simulink model "APP_MyApplication"  (R2018b)
settings: Solver=VariableStepDiscrete  StartTime=0.0  StopTime=10  RelTol=1e-3
PreLoadFcn:
  | if(exist('MBDS_ModelCallback', 'file')), MBDS_ModelCallback('PreLoad'); end;
PostLoadFcn:
  | if(exist('MBDS_ModelCallback', 'file')), MBDS_ModelCallback('PostLoad'); end;
InitFcn:
  | if(exist('MBDS_ModelCallback', 'file')), MBDS_ModelCallback('Init'); end;
StartFcn:
  | if(exist('MBDS_ModelCallback', 'file')), MBDS_ModelCallback('Start'); end;
StopFcn:
  | if(exist('MBDS_ModelCallback', 'file')), MBDS_ModelCallback('Stop'); end;
undefined symbols (not defined in the file): sigbuilder_block, Ts
libraries: KIBES_Signal x499, simulink x8
(part 7 of 10)

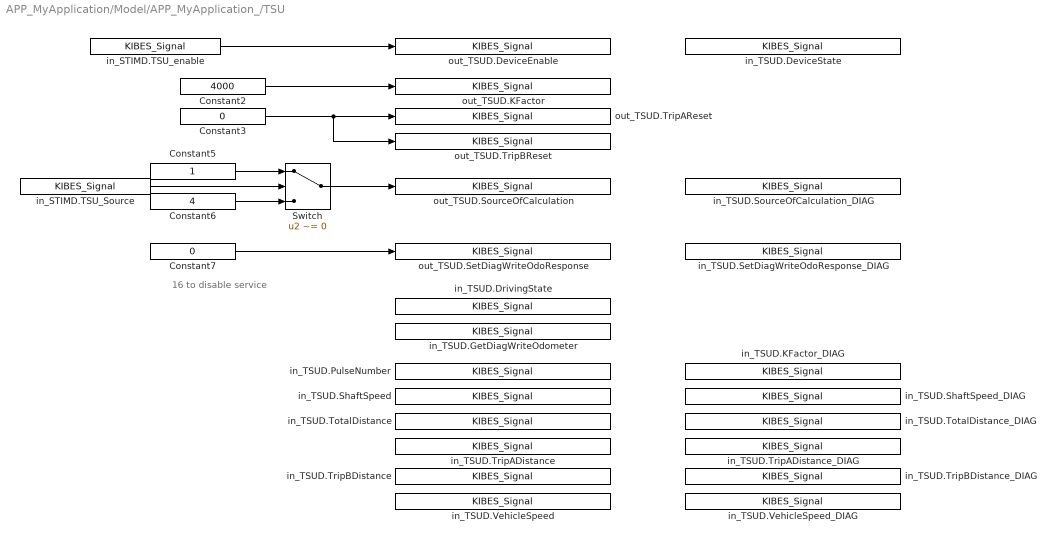
== system APP_MyApplication/Model/APP_MyApplication_/TSU ==
  note: 16 to disable service
  Constant2 : Constant  InitFcn=|  Value=4000  OutDataTypeStr=uint32
      | if(exist('MBDS_BlockCallback', 'file'))
      |    MBDS_BlockCallback('Update', gcb);  
      | end
  Constant3 : Constant  InitFcn=|  Value=0  OutDataTypeStr=boolean
      | if(exist('MBDS_BlockCallback', 'file'))
      |    MBDS_BlockCallback('Update', gcb);  
      | end
  Constant5 : Constant  InitFcn=|  OutDataTypeStr=uint8
      | if(exist('MBDS_BlockCallback', 'file'))
      |    MBDS_BlockCallback('Update', gcb);  
      | end
  Constant6 : Constant  InitFcn=|  Value=4  OutDataTypeStr=uint8
      | if(exist('MBDS_BlockCallback', 'file'))
      |    MBDS_BlockCallback('Update', gcb);  
      | end
  Constant7 : Constant  InitFcn=|  Value=0  OutDataTypeStr=uint8
      | if(exist('MBDS_BlockCallback', 'file'))
      |    MBDS_BlockCallback('Update', gcb);  
      | end
  Switch : Switch  InitFcn=|  Criteria=u2 ~= 0  OutDataTypeStr=Inherit: Inherit via back propagation  mask(Switch){MBDS_LibraryBlock=on, OutDataTypeStr_=Inherit: Inherit via back propagation, SaturateOnIntegerOverflow_=off, InputSameDT_=off, MBDS_BlockVersion=07.21.05}
      | if(exist('MBDS_BlockCallback', 'file'))
      |    MBDS_BlockCallback('Update', gcb);  
      | end
      mask prompts: MBDS_LibraryBlock "MBDS library block"; OutDataTypeStr_ "Output data type:"; SaturateOnIntegerOverflow_ "Saturate on integer overflow"; InputSameDT_ "Require all inputs to have the same data type"; MBDS_BlockVersion "Block version:"
      mask help: Pass through input 1 when input 2 is not equal to zero; otherwise pass through input 3. The inputs are numbered top to bottom (or left to right). The first and third input ports are data ports, and the second input port is the control port.
      mask init: same as APP_MyApplication/Model/APP_MyApplication_/OR
      mask Help: eval(['open([workdir(''library_dir:''),''\Blockset\help\'',get_param(gcb,''MaskType''),''.html''])'])
      mask TypeOptions OutDataTypeStr_: Inherit: Inherit via back propagation | single | int8 | uint8 | int16 | uint16 | int32 | uint32
      mask DialogControl ParameterTabVar0 Prompt: Signal Attributes
      mask DialogControl ParameterTabVar01 Prompt: Version
  in_STIMD.TSU_Source : KIBES_Signal/KIBES_Signal  MBDS_LibraryBlock=on  DatabaseKey=619  SignalName=STIMD.TSU_Source  SymbolName=STIMD_TSU_Source_000619  DataType=boolean  Init=0  Slope=1  Bias=0  DataSize=1  fpDataType=boolean  BlockIOType=Inport  DeviceType=2
  in_STIMD.TSU_enable : KIBES_Signal/KIBES_Signal  MBDS_LibraryBlock=on  DatabaseKey=391  SignalName=STIMD.TSU_enable  SymbolName=STIMD_TSU_enable_000391  DataType=boolean  Init=1  Slope=1  Bias=0  DataSize=1  fpDataType=boolean  BlockIOType=Inport  DeviceType=2
  in_TSUD.DeviceState : KIBES_Signal/KIBES_Signal  MBDS_LibraryBlock=on  DatabaseKey=379  SignalName=TSUD.DeviceState  SymbolName=TSUD_DeviceState_000379  DataType=uint16  Init=0  Slope=1  Bias=0  DataSize=1  fpDataType=uint16  BlockIOType=Inport  DeviceType=0
  in_TSUD.DrivingState : KIBES_Signal/KIBES_Signal  MBDS_LibraryBlock=on  DatabaseKey=376  SignalName=TSUD.DrivingState  SymbolName=TSUD_DrivingState_000376  DataType=boolean  Init=0  Slope=1  Bias=0  DataSize=1  fpDataType=boolean  BlockIOType=Inport  DeviceType=0
  in_TSUD.GetDiagWriteOdometer : KIBES_Signal/KIBES_Signal  MBDS_LibraryBlock=on  DatabaseKey=383  SignalName=TSUD.GetDiagWriteOdometer  SymbolName=TSUD_GetDiagWriteOdometer_000383  DataType=boolean  Init=0  Slope=1  Bias=0  DataSize=1  fpDataType=boolean  BlockIOType=Inport  DeviceType=0
  in_TSUD.KFactor_DIAG : KIBES_Signal/KIBES_Signal  MBDS_LibraryBlock=on  DatabaseKey=375  SignalName=TSUD.KFactor_DIAG  SymbolName=TSUD_KFactor_DIAG_000375  DataType=uint16  Init=1  Slope=1  Bias=0  DataSize=1  fpDataType=uint16  BlockIOType=Inport  DeviceType=0
  in_TSUD.PulseNumber : KIBES_Signal/KIBES_Signal  MBDS_LibraryBlock=on  DatabaseKey=381  SignalName=TSUD.PulseNumber  SymbolName=TSUD_PulseNumber_000381  DataType=uint16  Init=0  Slope=1  Bias=0  DataSize=1  fpDataType=uint16  BlockIOType=Inport  DeviceType=0
  in_TSUD.SetDiagWriteOdoResponse_DIAG : KIBES_Signal/KIBES_Signal  MBDS_LibraryBlock=on  DatabaseKey=374  SignalName=TSUD.SetDiagWriteOdoResponse_DIAG  SymbolName=TSUD_SetDiagWriteOdoResponse_DIAG_000374  DataType=uint16  Init=1  Slope=1  Bias=0  DataSize=1  fpDataType=uint16  BlockIOType=Inport  DeviceType=0
  in_TSUD.ShaftSpeed : KIBES_Signal/KIBES_Signal  MBDS_LibraryBlock=on  DatabaseKey=382  SignalName=TSUD.ShaftSpeed  SymbolName=TSUD_ShaftSpeed_000382  DataType=uint16  Init=0  Slope=1  Bias=0  DataSize=1  fpDataType=uint16  BlockIOType=Inport  DeviceType=0
  in_TSUD.ShaftSpeed_DIAG : KIBES_Signal/KIBES_Signal  MBDS_LibraryBlock=on  DatabaseKey=370  SignalName=TSUD.ShaftSpeed_DIAG  SymbolName=TSUD_ShaftSpeed_DIAG_000370  DataType=uint16  Init=1  Slope=1  Bias=0  DataSize=1  fpDataType=uint16  BlockIOType=Inport  DeviceType=0
  in_TSUD.SourceOfCalculation_DIAG : KIBES_Signal/KIBES_Signal  MBDS_LibraryBlock=on  DatabaseKey=369  SignalName=TSUD.SourceOfCalculation_DIAG  SymbolName=TSUD_SourceOfCalculation_DIAG_000369  DataType=uint16  Init=1  Slope=1  Bias=0  DataSize=1  fpDataType=uint16  BlockIOType=Inport  DeviceType=0
  in_TSUD.TotalDistance : KIBES_Signal/KIBES_Signal  MBDS_LibraryBlock=on  DatabaseKey=384  SignalName=TSUD.TotalDistance  SymbolName=TSUD_TotalDistance_000384  DataType=uint32  Init=0  Slope=1  Bias=0  DataSize=1  fpDataType=uint32  BlockIOType=Inport  DeviceType=0
  in_TSUD.TotalDistance_DIAG : KIBES_Signal/KIBES_Signal  MBDS_LibraryBlock=on  DatabaseKey=368  SignalName=TSUD.TotalDistance_DIAG  SymbolName=TSUD_TotalDistance_DIAG_000368  DataType=uint16  Init=1  Slope=1  Bias=0  DataSize=1  fpDataType=uint16  BlockIOType=Inport  DeviceType=0
  in_TSUD.TripADistance : KIBES_Signal/KIBES_Signal  MBDS_LibraryBlock=on  DatabaseKey=378  SignalName=TSUD.TripADistance  SymbolName=TSUD_TripADistance_000378  DataType=uint32  Init=0  Slope=1  Bias=0  DataSize=1  fpDataType=uint32  BlockIOType=Inport  DeviceType=0
  in_TSUD.TripADistance_DIAG : KIBES_Signal/KIBES_Signal  MBDS_LibraryBlock=on  DatabaseKey=372  SignalName=TSUD.TripADistance_DIAG  SymbolName=TSUD_TripADistance_DIAG_000372  DataType=uint16  Init=1  Slope=1  Bias=0  DataSize=1  fpDataType=uint16  BlockIOType=Inport  DeviceType=0
  in_TSUD.TripBDistance : KIBES_Signal/KIBES_Signal  MBDS_LibraryBlock=on  DatabaseKey=377  SignalName=TSUD.TripBDistance  SymbolName=TSUD_TripBDistance_000377  DataType=uint32  Init=0  Slope=1  Bias=0  DataSize=1  fpDataType=uint32  BlockIOType=Inport  DeviceType=0
  in_TSUD.TripBDistance_DIAG : KIBES_Signal/KIBES_Signal  MBDS_LibraryBlock=on  DatabaseKey=373  SignalName=TSUD.TripBDistance_DIAG  SymbolName=TSUD_TripBDistance_DIAG_000373  DataType=uint16  Init=1  Slope=1  Bias=0  DataSize=1  fpDataType=uint16  BlockIOType=Inport  DeviceType=0
  in_TSUD.VehicleSpeed : KIBES_Signal/KIBES_Signal  MBDS_LibraryBlock=on  DatabaseKey=380  SignalName=TSUD.VehicleSpeed  SymbolName=TSUD_VehicleSpeed_000380  DataType=uint16  Init=0  Slope=1  Bias=0  DataSize=1  fpDataType=uint16  BlockIOType=Inport  DeviceType=0
  in_TSUD.VehicleSpeed_DIAG : KIBES_Signal/KIBES_Signal  MBDS_LibraryBlock=on  DatabaseKey=371  SignalName=TSUD.VehicleSpeed_DIAG  SymbolName=TSUD_VehicleSpeed_DIAG_000371  DataType=uint16  Init=1  Slope=1  Bias=0  DataSize=1  fpDataType=uint16  BlockIOType=Inport  DeviceType=0
  out_TSUD.DeviceEnable : KIBES_Signal/KIBES_Signal  MBDS_LibraryBlock=on  DatabaseKey=385  SignalName=TSUD.DeviceEnable  SymbolName=TSUD_DeviceEnable_000385  DataType=boolean  Init=0  Slope=1  Bias=0  DataSize=1  fpDataType=boolean  BlockIOType=Outport  DeviceType=0
  out_TSUD.KFactor : KIBES_Signal/KIBES_Signal  MBDS_LibraryBlock=on  DatabaseKey=387  SignalName=TSUD.KFactor  SymbolName=TSUD_KFactor_000387  DataType=uint32  Init=0  Slope=1  Bias=0  DataSize=1  fpDataType=uint32  BlockIOType=Outport  DeviceType=0
  out_TSUD.SetDiagWriteOdoResponse : KIBES_Signal/KIBES_Signal  MBDS_LibraryBlock=on  DatabaseKey=386  SignalName=TSUD.SetDiagWriteOdoResponse  SymbolName=TSUD_SetDiagWriteOdoResponse_000386  DataType=uint8  Init=0  Slope=1  Bias=0  DataSize=1  fpDataType=uint8  BlockIOType=Outport  DeviceType=0
  out_TSUD.SourceOfCalculation : KIBES_Signal/KIBES_Signal  MBDS_LibraryBlock=on  DatabaseKey=390  SignalName=TSUD.SourceOfCalculation  SymbolName=TSUD_SourceOfCalculation_000390  DataType=uint8  Init=0  Slope=1  Bias=0  DataSize=1  fpDataType=uint8  BlockIOType=Outport  DeviceType=0
  out_TSUD.TripAReset : KIBES_Signal/KIBES_Signal  MBDS_LibraryBlock=on  DatabaseKey=388  SignalName=TSUD.TripAReset  SymbolName=TSUD_TripAReset_000388  DataType=boolean  Init=0  Slope=1  Bias=0  DataSize=1  fpDataType=boolean  BlockIOType=Outport  DeviceType=0
  out_TSUD.TripBReset : KIBES_Signal/KIBES_Signal  MBDS_LibraryBlock=on  DatabaseKey=389  SignalName=TSUD.TripBReset  SymbolName=TSUD_TripBReset_000389  DataType=boolean  Init=0  Slope=1  Bias=0  DataSize=1  fpDataType=boolean  BlockIOType=Outport  DeviceType=0
  wires:
  Constant2/1 -> out_TSUD.KFactor/1
  Constant3/1 -> out_TSUD.TripBReset/1, out_TSUD.TripAReset/1
  Switch/1 -> out_TSUD.SourceOfCalculation/1
  Constant5/1 -> Switch/1
  Constant6/1 -> Switch/3
  in_STIMD.TSU_Source/1 -> Switch/2
  Constant7/1 -> out_TSUD.SetDiagWriteOdoResponse/1
  in_STIMD.TSU_enable/1 -> out_TSUD.DeviceEnable/1

== system APP_MyApplication/Model/APP_MyApplication_/TimerPulse ==
  note: Timer Pulse
  bo_Enable : Inport  OutDataTypeStr=boolean
  EdgeRising : Subsystem  InitFcn=|  mask(EdgeRising){MBDS_LibraryBlock=on, R_Enabled=off, IV_Enabled=off, IV=0, MBDS_BlockVersion=05.32}
      | if(exist('MBDS_BlockCallback', 'file'))
      |    MBDS_BlockCallback('Update', gcb);
      | end
      mask prompts: MBDS_LibraryBlock "MBDS library block"; R_Enabled "Show R port"; IV_Enabled "Show IV port"; IV "Initial value (IV):"; MBDS_BlockVersion "Block version:"
      mask help: The output indicates true if the input value changes from false to true.
      mask init: same as APP_MyApplication/Model/APP_MyApplication_/OR
      mask Help: eval(['open([workdir(''library_dir:''),''\Blockset\help\'',get_param(gcb,''MaskType''),''.html''])'])
      mask Callback R_Enabled:
      | % Update mask parameter dialog
      | if(exist('MBDS_BlockCallback', 'file'))
      |    MBDS_BlockCallback('R_Enabled', gcb);
      | end
      mask Callback IV_Enabled:
      | % Update mask parameter dialog
      | if(exist('MBDS_BlockCallback', 'file'))
      |    MBDS_BlockCallback('IV_Enabled', gcb);
      | end
      mask Callback IV:
      | % Adopt Value
      | if(exist('MBDS_BlockCallback', 'file'))
      |    MBDS_BlockCallback('IV', gcb);
      | end
      mask DialogControl ParameterTabVar0 Prompt: Main
      mask DialogControl ParameterTabVar01 Prompt: Version
      mask Display:
      | % Show icon or block text
      | if(exist('EdgeRising.tif', 'file'))
      |    image('EdgeRising.tif', [0.295739348370927 0.17 0.378947368421053 0.66]);
      |    disp('')
      | else
      |    disp(sprintf('Rising\nEdge\nDetection'));
      | end
      | 
      | % Display port labels
      | port_label('input', 1, 'u');
      | port_label('output', 1, 'y');
  TimeSource : Subsystem  InitFcn=|  mask(TimeSource){MBDS_LibraryBlock=on, InputValue=5s, MBDS_BlockVersion=07.21.04}
      | if(exist('MBDS_BlockCallback', 'file'))
      |    MBDS_BlockCallback('Update', gcb);
      | end
      mask prompts: MBDS_LibraryBlock "MBDS Library Block"; InputValue "Constant value:"; MBDS_BlockVersion "Block version:"
      mask help: This block outputs a constant time signal based on a uint32 data type. Specify the time by the 'Constant value' parameter. Comply to the format: 1d2h3m4s5ms, for example 12d10h34m4s231ms, 1s500ms or 2h1s.
      mask init:
      | MBDS_BlockCallback('Copy', gcb);
      | Text = InputValue;
      | try
      |    % Try to evaluate project constant 
      |    EvalValue = evalin('base', InputValue);
      |    if(~isempty(EvalValue))
      |       InputValue = EvalValue;
      |    end
      | end
      | % Convert string to value (enable silent mode)
      | Value = ConvertSignalValue(InputValue, 'time', 'Str2Val', true);
      mask Help: eval(['open([workdir(''Library_Dir:''),''\Blockset\Help\'',get_param(gcb,''MaskType''),''.html''])'])
      mask DialogControl ParameterTabVar0 Prompt: Main
      mask DialogControl ParameterTabVar01 Prompt: Version
      mask Display: disp([' ',Text,' ']);
  Timer_RE1 : Subsystem  InitFcn=|  mask(Timer_RE){MBDS_LibraryBlock=on, dT_Enabled=off, dT=1000*Ts, E_Enabled=off, R_Enabled=on, IV_Enabled=on, IV=0, y_Enabled=on, x_Enabled=off, OutDataTypeStr=Inherit: Inherit via back propagation, MBDS_BlockVersion=05.20}
      | if(exist('MBDS_BlockCallback', 'file'))
      |    MBDS_BlockCallback('Update', gcb);
      | end
      mask prompts: MBDS_LibraryBlock "MBDS library block"; dT_Enabled "Show dT port"; dT "Sample rate (dT):"; E_Enabled "Show E port"; R_Enabled "Show R port"; IV_Enabled "Show IV port"; IV "Initial value (IV):"; y_Enabled "Show y port"; x_Enabled "Show x port"; OutDataTypeStr "Output data type:"; MBDS_BlockVersion "Block version:"
      mask help: The block indicates true, if the initial time IV has not passed since the last reset of the block. Reset can only be performed, if the counter has run down to zero.
      mask init: same as APP_MyApplication/Model/APP_MyApplication_/OR
      settings: AttributesFormatString=dT = %<dT>
      mask Help: eval(['open([workdir(''library_dir:''),''\Blockset\help\'',get_param(gcb,''MaskType''),''.html''])'])
      mask Callback dT_Enabled:
      | % Update mask parameter dialog
      | if(exist('MBDS_BlockCallback', 'file'))
      |    MBDS_BlockCallback('dT_Enabled', gcb);
      | end
      mask Callback dT:
      | % Adopt Value
      | if(exist('MBDS_BlockCallback', 'file'))
      |    MBDS_BlockCallback('dT', gcb);
      | end
      mask Callback R_Enabled:
      | % Update mask parameter dialog
      | if(exist('MBDS_BlockCallback', 'file'))
      |    MBDS_BlockCallback('R_Enabled', gcb);
      | end
      mask Callback IV_Enabled:
      | % Update mask parameter dialog
      | if(exist('MBDS_BlockCallback', 'file'))
      |    MBDS_BlockCallback('IV_Enabled', gcb);
      | end
      mask Callback IV:
      | % Adopt Value
      | if(exist('MBDS_BlockCallback', 'file'))
      |    MBDS_BlockCallback('IV', gcb);
      | end
      mask Callback y_Enabled:
      | % Update mask parameter dialog
      | if(exist('MBDS_BlockCallback', 'file'))
      |    MBDS_BlockCallback('y_Enabled', gcb);
      | end
      mask Callback x_Enabled:
      | % Update mask parameter dialog
      | if(exist('MBDS_BlockCallback', 'file'))
      |    MBDS_BlockCallback('x_Enabled', gcb);
      | end
      mask TypeOptions OutDataTypeStr: Inherit: Inherit via back propagation | int8 | uint8 | int16 | uint16 | int32 | uint32
      mask Callback OutDataTypeStr:
      | % Configure data type
      | if(exist('MBDS_BlockCallback', 'file'))
      |    MBDS_BlockCallback('OutDataTypeStr', gcb);
      | end
      mask DialogControl ParameterTabVar0 Prompt: Main
      mask DialogControl ParameterTabVar01 Prompt: Signal Attributes
      mask DialogControl ParameterTabVar012 Prompt: Version
      mask Display:
      | % Show icon or block text
      | if(exist('Timer.tif', 'file'))
      |    image('Timer.tif', [0.295739348370927 0.17 0.378947368421053 0.66]);
      |    disp('')
      | else
      |    disp(sprintf('Timer'));
      | end
      | 
      | % Display port labels
      | port_label('input', 1, 'R');
      | port_label('input', 2, 'IV');
      | port_label('output', 1, 'y');
  bo_Pulse : Outport
  wires:
  EdgeRising/1(y) -> Timer_RE1/1(R)
  Timer_RE1/1(y) -> bo_Pulse/1
  bo_Enable/1 -> EdgeRising/1(u)
  TimeSource/1(Out) -> Timer_RE1/2(IV)

== system APP_MyApplication/Model/APP_MyApplication_/UDS Service ==
  note: array
  note: IOControl: RAM device signal to access via IOControl DID F010, Read in all sessions, Write in Extended L3
  note: Stop 31 02 02 00
  note: Start: 31 01 02 00
  note: Request Result 31 03 02 00 -> response is set in u8Response
  note: END
  Chart : Stateflow chart  TreatAsAtomicUnit=on
      settings: CopyFcn=|
      | if(exist('MBDS_BlockCallback', 'file'))
      |    MBDS_BlockCallback('Copy', gcb);
      | end
  Constant : Constant  InitFcn=|  OutDataTypeStr=uint8
      | if(exist('MBDS_BlockCallback', 'file'))
      |    MBDS_BlockCallback('Update', gcb);  
      | end
  Constant1 : Constant  InitFcn=|  Value=2  OutDataTypeStr=uint16
      | if(exist('MBDS_BlockCallback', 'file'))
      |    MBDS_BlockCallback('Update', gcb);  
      | end
  Constant2 : Constant  InitFcn=|  Value=3  OutDataTypeStr=uint32
      | if(exist('MBDS_BlockCallback', 'file'))
      |    MBDS_BlockCallback('Update', gcb);  
      | end
  Constant3 : Constant  InitFcn=|  Value=15  OutDataTypeStr=uint8
      | if(exist('MBDS_BlockCallback', 'file'))
      |    MBDS_BlockCallback('Update', gcb);  
      | end
  Constant4 : Constant  InitFcn=|  Value=33  OutDataTypeStr=uint8
      | if(exist('MBDS_BlockCallback', 'file'))
      |    MBDS_BlockCallback('Update', gcb);  
      | end
  Constant5 : Constant  InitFcn=|  Value=0  OutDataTypeStr=uint8
      | if(exist('MBDS_BlockCallback', 'file'))
      |    MBDS_BlockCallback('Update', gcb);  
      | end
  RSFlipFlop : Subsystem  InitFcn=|  mask(RSFlipFlop){MBDS_LibraryBlock=on, Q_Enabled=on, Not_Q_Enabled=on, MBDS_BlockVersion=08.20.02}
      | if(exist('MBDS_BlockCallback', 'file'))
      |    MBDS_BlockCallback('Update', gcb);
      | end
      mask prompts: MBDS_LibraryBlock "MBDS library block"; Q_Enabled "Show Q port"; Not_Q_Enabled "Show ~Q port"; MBDS_BlockVersion "Block version:"
      mask help: A flip flop. The reset input (RST) dominates the set input (SET).
      mask init: same as APP_MyApplication/Model/APP_MyApplication_/OR
      mask Help: eval(['open([workdir(''library_dir:''),''\Blockset\help\'',get_param(gcb,''MaskType''),''.html''])'])
      mask Callback Q_Enabled:
      | % Update mask parameter dialog
      | if(exist('MBDS_BlockCallback', 'file'))
      |    MBDS_BlockCallback('Q_Enabled', gcb);
      | end
      mask Callback Not_Q_Enabled:
      | % Update mask parameter dialog
      | if(exist('MBDS_BlockCallback', 'file'))
      |    MBDS_BlockCallback('Not_Q_Enabled', gcb);
      | end
      mask DialogControl ParameterTabVar0 Prompt: Main
      mask DialogControl ParameterTabVar01 Prompt: Version
      mask Display:
      | % Show icon or block text
      | if(exist('RSFlipFlop.tif', 'file'))
      |    image('RSFlipFlop.tif', [0.295739348370927 0.17 0.378947368421053 0.66]);
      |    disp('')
      | else
      |    disp(sprintf('RS\nFlipFlop'));
      | end
      | 
      | % Display port labels
      | port_label('input', 1, 'SET');
      | port_label('input', 2, 'RST');
      | port_label('output', 1, 'Q');
      | port_label('output', 2, '~Q');
  Switch5 : Switch  InitFcn=|  Criteria=u2 ~= 0  OutDataTypeStr=Inherit: Inherit via back propagation  mask(Switch){MBDS_LibraryBlock=on, OutDataTypeStr_=Inherit: Inherit via back propagation, SaturateOnIntegerOverflow_=off, InputSameDT_=off, MBDS_BlockVersion=07.21.05}
      | if(exist('MBDS_BlockCallback', 'file'))
      |    MBDS_BlockCallback('Update', gcb);  
      | end
      mask prompts: MBDS_LibraryBlock "MBDS library block"; OutDataTypeStr_ "Output data type:"; SaturateOnIntegerOverflow_ "Saturate on integer overflow"; InputSameDT_ "Require all inputs to have the same data type"; MBDS_BlockVersion "Block version:"
      mask help: Pass through input 1 when input 2 is not equal to zero; otherwise pass through input 3. The inputs are numbered top to bottom (or left to right). The first and third input ports are data ports, and the second input port is the control port.
      mask init: same as APP_MyApplication/Model/APP_MyApplication_/OR
      mask Help: eval(['open([workdir(''library_dir:''),''\Blockset\help\'',get_param(gcb,''MaskType''),''.html''])'])
      mask TypeOptions OutDataTypeStr_: Inherit: Inherit via back propagation | single | int8 | uint8 | int16 | uint16 | int32 | uint32
      mask DialogControl ParameterTabVar0 Prompt: Signal Attributes
      mask DialogControl ParameterTabVar01 Prompt: Version
  in_DigitalInputs.IN_DIG_39 : KIBES_Signal/KIBES_Signal  MBDS_LibraryBlock=on  DatabaseKey=487  SignalName=DigitalInputs.IN_DIG_39  SymbolName=DigitalInputs_IN_DIG_39_000487  DataType=boolean  Init=0  Slope=1  Bias=0  DataSize=1  fpDataType=boolean  BlockIOType=Inport  DeviceType=0
  in_UDSServices.RoutineControlService.RoutineCtrl1.RequestRoutineResults : KIBES_Signal/KIBES_Signal  MBDS_LibraryBlock=on  DatabaseKey=613  SignalName=UDSServices.RoutineControlService.RoutineCtrl1.RequestRoutineResults  SymbolName=UDSServices_RoutineControlService_RoutineCtrl1_RequestR_000613  DataType=boolean  Init=0  Slope=1  Bias=0  DataSize=1  fpDataType=boolean  BlockIOType=Inport  DeviceType=0
  in_UDSServices.RoutineControlService.RoutineCtrl1.StartRoutine : KIBES_Signal/KIBES_Signal  MBDS_LibraryBlock=on  DatabaseKey=615  SignalName=UDSServices.RoutineControlService.RoutineCtrl1.StartRoutine  SymbolName=UDSServices_RoutineControlService_RoutineCtrl1_StartRou_000615  DataType=boolean  Init=0  Slope=1  Bias=0  DataSize=1  fpDataType=boolean  BlockIOType=Inport  DeviceType=0
  in_UDSServices.RoutineControlService.RoutineCtrl1.StopRoutine : KIBES_Signal/KIBES_Signal  MBDS_LibraryBlock=on  DatabaseKey=616  SignalName=UDSServices.RoutineControlService.RoutineCtrl1.StopRoutine  SymbolName=UDSServices_RoutineControlService_RoutineCtrl1_StopRout_000616  DataType=boolean  Init=0  Slope=1  Bias=0  DataSize=1  fpDataType=boolean  BlockIOType=Inport  DeviceType=0
  in_UDSServices.RoutineControlService.RoutineCtrl1.u8Response : KIBES_Signal/KIBES_Signal  MBDS_LibraryBlock=on  DatabaseKey=617  SignalName=UDSServices.RoutineControlService.RoutineCtrl1.u8Response  SymbolName=UDSServices_RoutineControlService_RoutineCtrl1_u8Respon_000617  DataType=uint8  Init=0  Slope=1  Bias=0  DataSize=1  fpDataType=uint8  BlockIOType=Inport  DeviceType=0
  out_RAMDevice.RAMDevice_udint : KIBES_Signal/KIBES_Signal  MBDS_LibraryBlock=on  DatabaseKey=609  SignalName=RAMDevice.RAMDevice_udint  SymbolName=RAMDevice_RAMDevice_udint_000609  DataType=uint32  Init=0  Slope=1  Bias=0  DataSize=1  fpDataType=uint32  BlockIOType=Outport  DeviceType=0
  out_RAMDevice.RAMDevice_uint : KIBES_Signal/KIBES_Signal  MBDS_LibraryBlock=on  DatabaseKey=610  SignalName=RAMDevice.RAMDevice_uint  SymbolName=RAMDevice_RAMDevice_uint_000610  DataType=uint16  Init=0  Slope=1  Bias=0  DataSize=1  fpDataType=uint16  BlockIOType=Outport  DeviceType=0
  out_RAMDevice.RAMDevice_usint : KIBES_Signal/KIBES_Signal  MBDS_LibraryBlock=on  DatabaseKey=611  SignalName=RAMDevice.RAMDevice_usint  SymbolName=RAMDevice_RAMDevice_usint_000611  DataType=uint8  Init=0  Slope=1  Bias=0  DataSize=1  fpDataType=uint8  BlockIOType=Outport  DeviceType=0
  out_RAMDevice.RoutineCtrl_Response : KIBES_Signal/KIBES_Signal  MBDS_LibraryBlock=on  DatabaseKey=618  SignalName=RAMDevice.RoutineCtrl_Response  SymbolName=RAMDevice_RoutineCtrl_Response_000618  DataType=uint8  Init=0  Slope=1  Bias=0  DataSize=1  fpDataType=uint8  BlockIOType=Outport  DeviceType=0
  out_UDSServices.RejectDiagnosticAccess : KIBES_Signal/KIBES_Signal  MBDS_LibraryBlock=on  DatabaseKey=608  SignalName=UDSServices.RejectDiagnosticAccess  SymbolName=UDSServices_RejectDiagnosticAccess_000608  DataType=boolean  Init=0  Slope=1  Bias=0  DataSize=1  fpDataType=boolean  BlockIOType=Outport  DeviceType=0
  out_UDSServices.RoutineControlService.RoutineCtrl1.ResponseCode : KIBES_Signal/KIBES_Signal  MBDS_LibraryBlock=on  DatabaseKey=614  SignalName=UDSServices.RoutineControlService.RoutineCtrl1.ResponseCode  SymbolName=UDSServices_RoutineControlService_RoutineCtrl1_Response_000614  DataType=uint8  Init=0  Slope=1  Bias=0  DataSize=1  fpDataType=uint8  BlockIOType=Outport  DeviceType=0
  wires:
  in_DigitalInputs.IN_DIG_39/1 -> out_UDSServices.RejectDiagnosticAccess/1
  Constant/1 -> out_RAMDevice.RAMDevice_usint/1
  Constant1/1 -> out_RAMDevice.RAMDevice_uint/1
  Constant2/1 -> out_RAMDevice.RAMDevice_udint/1
  in_UDSServices.RoutineControlService.RoutineCtrl1.StartRoutine/1 -> Chart/1(boRequest), RSFlipFlop/1(SET)
  in_UDSServices.RoutineControlService.RoutineCtrl1.StopRoutine/1 -> RSFlipFlop/2(RST)
  RSFlipFlop/1(Q) -> Switch5/2
  Constant3/1 -> Switch5/1
  Constant4/1 -> Switch5/3
  Switch5/1 -> out_UDSServices.RoutineControlService.RoutineCtrl1.ResponseCode/1
  Constant5/1 -> Chart/2(u8Return)
  Chart/1(u8Response) -> out_RAMDevice.RoutineCtrl_Response/1

== system APP_MyApplication/Outputs/AnalyseOutputs/AND ==
  note: AND
  u1 : Inport  OutDataTypeStr=boolean
  u2 : Inport  Port=2  OutDataTypeStr=boolean
  DataType : DataTypeConversion  OutDataTypeStr=boolean  SaturateOnIntegerOverflow=on
  Operator : Logic  AllPortsSameDT=off  OutDataTypeStr=boolean
  y : Outport
  wires:
  Operator/1 -> DataType/1
  u1/1 -> Operator/1
  u2/1 -> Operator/2
  DataType/1 -> y/1

== system APP_MyApplication/Outputs/AnalyseOutputs/LE1 ==
  note: LE
  u1 : Inport
  u2 : Inport  Port=2
  Operator : RelationalOperator  Operator=<=  OutDataTypeStr=boolean  RndMeth=Nearest  InputSameDT=on
  y : Outport
  wires:
  Operator/1 -> y/1
  u2/1 -> Operator/2
  u1/1 -> Operator/1

== system APP_MyApplication/Outputs/AnalyseOutputs/LE2 ==
  note: LE
  u1 : Inport
  u2 : Inport  Port=2
  Operator : RelationalOperator  Operator=<=  OutDataTypeStr=boolean  RndMeth=Nearest  InputSameDT=on
  y : Outport
  wires:
  Operator/1 -> y/1
  u2/1 -> Operator/2
  u1/1 -> Operator/1

== system APP_MyApplication/Model/APP_MyApplication_/D-CAN(1)/NOT ==
  note: NOT
  u1 : Inport  OutDataTypeStr=boolean
  DataType : DataTypeConversion  OutDataTypeStr=boolean
  Operator : Logic  Operator=NOT  Inputs=1  AllPortsSameDT=off  OutDataTypeStr=boolean
  y : Outport
  wires:
  Operator/1 -> DataType/1
  u1/1 -> Operator/1
  DataType/1 -> y/1

== system APP_MyApplication/Model/APP_MyApplication_/DM13/OR1 ==
  note: OR
  u1 : Inport  OutDataTypeStr=boolean
  u2 : Inport  Port=2  OutDataTypeStr=boolean
  DataType : DataTypeConversion  OutDataTypeStr=boolean
  Operator : Logic  Operator=OR  AllPortsSameDT=off  OutDataTypeStr=boolean
  y : Outport
  wires:
  Operator/1 -> DataType/1
  u1/1 -> Operator/1
  u2/1 -> Operator/2
  DataType/1 -> y/1

== system APP_MyApplication/Model/APP_MyApplication_/DM2_3_11/OR1 ==
  note: OR
  u1 : Inport  OutDataTypeStr=boolean
  u2 : Inport  Port=2  OutDataTypeStr=boolean
  DataType : DataTypeConversion  OutDataTypeStr=boolean
  Operator : Logic  Operator=OR  AllPortsSameDT=off  OutDataTypeStr=boolean
  y : Outport
  wires:
  Operator/1 -> DataType/1
  u1/1 -> Operator/1
  u2/1 -> Operator/2
  DataType/1 -> y/1

== system APP_MyApplication/Model/APP_MyApplication_/DM2_3_11/OR2 ==
  note: OR
  u1 : Inport  OutDataTypeStr=boolean
  u2 : Inport  Port=2  OutDataTypeStr=boolean
  DataType : DataTypeConversion  OutDataTypeStr=boolean
  Operator : Logic  Operator=OR  AllPortsSameDT=off  OutDataTypeStr=boolean
  y : Outport
  wires:
  Operator/1 -> DataType/1
  u1/1 -> Operator/1
  u2/1 -> Operator/2
  DataType/1 -> y/1

== system APP_MyApplication/Model/APP_MyApplication_/DM2_3_11/OR3 ==
  note: OR
  u1 : Inport  OutDataTypeStr=boolean
  u2 : Inport  Port=2  OutDataTypeStr=boolean
  DataType : DataTypeConversion  OutDataTypeStr=boolean
  Operator : Logic  Operator=OR  AllPortsSameDT=off  OutDataTypeStr=boolean
  y : Outport
  wires:
  Operator/1 -> DataType/1
  u1/1 -> Operator/1
  u2/1 -> Operator/2
  DataType/1 -> y/1

== system APP_MyApplication/Model/APP_MyApplication_/DM4RX/EQ ==
  note: EQ
  u1 : Inport
  u2 : Inport  Port=2
  Operator : RelationalOperator  Operator===  OutDataTypeStr=boolean  RndMeth=Nearest  InputSameDT=on
  y : Outport
  wires:
  Operator/1 -> y/1
  u1/1 -> Operator/1
  u2/1 -> Operator/2

== system APP_MyApplication/Model/APP_MyApplication_/DM4RX/SRFlipFlop ==
  note: SRFlipFlop
  SET : Inport  OutDataTypeStr=boolean
  RST : Inport  Port=2  OutDataTypeStr=boolean
  Constant : Constant  Value=0  OutDataTypeStr=Inherit: Inherit via back propagation
  Constant1 : Constant  OutDataTypeStr=Inherit: Inherit via back propagation
  Data Type Duplicate : DataTypeDuplicate  NumInputPorts=3
  Logical Operator : Logic  Operator=NOT  AllPortsSameDT=off  OutDataTypeStr=boolean
  Switch1 : Switch  Criteria=u2 ~= 0  OutDataTypeStr=Inherit: Inherit via back propagation
  Switch2 : Switch  Criteria=u2 ~= 0  OutDataTypeStr=Inherit: Inherit via back propagation
  Unit Delay : UnitDelay  SampleTime=-1
  ~Q : Terminator
  Q : Outport
  wires:
  Switch1/1 -> Q/1, Data Type Duplicate/3, Unit Delay/1, Logical Operator/1
  Switch2/1 -> Switch1/3
  Logical Operator/1 -> ~Q/1
  Unit Delay/1 -> Switch2/3
  SET/1 -> Data Type Duplicate/2, Switch1/2
  Constant1/1 -> Switch1/1
  Constant/1 -> Switch2/1
  RST/1 -> Data Type Duplicate/1, Switch2/2

== system APP_MyApplication/Model/APP_MyApplication_/DTC/DateTimeDisassemble ==
  note: Output
  note: Maximum
  note: Current
  note: Add 1970 years
  note: DateTimeDisassemble
  DT : Inport  OutDataTypeStr=uint32
  Add : Sum  OutDataTypeStr=uint32
  Add1 : Sum  OutDataTypeStr=uint16
  Add4 : Sum  OutDataTypeStr=uint8
  Bus Creator : BusCreator  Inputs='u8_Seconds','u8_Minutes','u8_Hours','u8_Day','u8_Month','u16_Year','u8_DayOfWeek'
  Bus Creator1 : BusCreator  Inputs=7
  Bus Selector : BusSelector  OutputSignals=u8_Seconds,u8_Minutes,u8_Hours,u8_Day,u8_Month,u16_Year,u8_DayOfWeek
  CheckIfTimeDataIsValid : Subsystem
  CheckLeapYearsAndRemainingDays : Subsystem
  Constant : Constant  OutDataTypeStr=uint8
  Constant1 : Constant  Value=1970  OutDataTypeStr=uint16
  Constant10 : Constant  Value=2099  OutDataTypeStr=uint16
  Constant11 : Constant  Value=12  OutDataTypeStr=uint8
  Constant12 : Constant  Value=31  OutDataTypeStr=uint8
  Constant13 : Constant  Value=4  OutDataTypeStr=uint8
  Constant7 : Constant  Value=59  OutDataTypeStr=uint8
  Constant8 : Constant  Value=59  OutDataTypeStr=uint8
  Constant9 : Constant  Value=23  OutDataTypeStr=uint8
  ConvertToDayOfWeek : Subsystem
  ConvertToMonthAndDay : Subsystem  TreatAsAtomicUnit=on
  ConvertToTimeAndNrOfDays : Subsystem
  Data Type Conversion1 : DataTypeConversion  OutDataTypeStr=uint8
  Switch : Switch  Criteria=u2 ~= 0
  Year : Outport  OutDataTypeStr=uint16
  Month : Outport  Port=2  OutDataTypeStr=uint8
  Day : Outport  Port=3  OutDataTypeStr=uint8
  Hours : Outport  Port=4  OutDataTypeStr=uint8
  Minutes : Outport  Port=5  OutDataTypeStr=uint8
  Seconds : Outport  Port=6  OutDataTypeStr=uint8
  DayOfWeek : Outport  Port=7  OutDataTypeStr=uint8
  ENO : Outport  Port=8  OutDataTypeStr=boolean
  wires:
  Add1/1 -> Bus Creator/6  "u16_Year"
  ConvertToTimeAndNrOfDays/1(u8_Seconds) -> Bus Creator/1  "u8_Seconds"
  ConvertToTimeAndNrOfDays/3(u8_Hours) -> Bus Creator/3  "u8_Hours"
  ConvertToTimeAndNrOfDays/2(u8_Minutes) -> Bus Creator/2  "u8_Minutes"
  ConvertToMonthAndDay/2(u16_DayMinusOne) -> Add/1
  CheckLeapYearsAndRemainingDays/2(u16_Year) -> Add1/1
  Constant1/1 -> Add1/2
  CheckLeapYearsAndRemainingDays/3(bo_LeapYear) -> ConvertToMonthAndDay/2(bo_LeapYear)
  DT/1 -> CheckIfTimeDataIsValid/1(u32_DateTime), ConvertToTimeAndNrOfDays/1(u32_DateTime)
  Add/1 -> Data Type Conversion1/1
  ConvertToMonthAndDay/1(u8_MonthMinusOne) -> Add4/1
  Add4/1 -> Bus Creator/5  "u8_Month"
  Bus Selector/1 -> Seconds/1  "<u8_Seconds>"
  Bus Selector/2 -> Minutes/1  "<u8_Minutes>"
  Bus Selector/3 -> Hours/1  "<u8_Hours>"
  Bus Selector/5 -> Month/1  "<u8_Month>"
  Bus Creator/1 -> Switch/1  "st_CurrDateTime"
  Switch/1 -> Bus Selector/1  "st_OutDateTime"
  Bus Creator1/1 -> Switch/3  "st_MaxDataTime"
  Constant7/1 -> Bus Creator1/1  "u8_Seconds"
  Constant8/1 -> Bus Creator1/2  "u8_Minutes"
  Constant9/1 -> Bus Creator1/3  "u8_Hours"
  Constant11/1 -> Bus Creator1/5  "u8_Month"
  Constant13/1 -> Bus Creator1/7  "u8_DayOfWeek"
  Bus Selector/4 -> Day/1  "<u8_Day>"
  Data Type Conversion1/1 -> Bus Creator/4  "u8_Day"
  Bus Selector/6 -> Year/1  "<u16_Year>"
  Constant12/1 -> Bus Creator1/4  "u8_Day"
  Constant10/1 -> Bus Creator1/6  "u16_Year"
  Bus Selector/7 -> DayOfWeek/1  "<u8_DayOfWeek>"
  ConvertToTimeAndNrOfDays/4(u16_NrOfDays) -> ConvertToDayOfWeek/1(u16_NrOfDays), CheckLeapYearsAndRemainingDays/1(u16_NrOfDays)
  Constant/1 -> Add4/2, Add/2
  ConvertToDayOfWeek/1(u8_DayOfWeek) -> Bus Creator/7  "u8_DayOfWeek"
  CheckLeapYearsAndRemainingDays/1(u16_TempDate) -> ConvertToMonthAndDay/1(u16_TempDate)
  CheckIfTimeDataIsValid/1(bo_ENO) -> ENO/1, Switch/2

== system APP_MyApplication/Model/APP_MyApplication_/DTC/GetBit ==
  note: GetBit
  u : Inport
  SEL : Inport  Port=2
  LoopOverBits : Subsystem
  y : Outport
  wires:
  u/1 -> LoopOverBits/1(u)
  SEL/1 -> LoopOverBits/2(SEL)
  LoopOverBits/1(y) -> y/1

== system APP_MyApplication/Model/APP_MyApplication_/DTC/GetBit1 ==
  note: GetBit
  u : Inport
  SEL : Inport  Port=2
  LoopOverBits : Subsystem
  y : Outport
  wires:
  u/1 -> LoopOverBits/1(u)
  SEL/1 -> LoopOverBits/2(SEL)
  LoopOverBits/1(y) -> y/1

== system APP_MyApplication/Model/APP_MyApplication_/DTC/GetBit2 ==
  note: GetBit
  u : Inport
  SEL : Inport  Port=2
  LoopOverBits : Subsystem
  y : Outport
  wires:
  u/1 -> LoopOverBits/1(u)
  SEL/1 -> LoopOverBits/2(SEL)
  LoopOverBits/1(y) -> y/1

== system APP_MyApplication/Model/APP_MyApplication_/DTC/GetBit3 ==
  note: GetBit
  u : Inport
  SEL : Inport  Port=2
  LoopOverBits : Subsystem
  y : Outport
  wires:
  u/1 -> LoopOverBits/1(u)
  SEL/1 -> LoopOverBits/2(SEL)
  LoopOverBits/1(y) -> y/1

== system APP_MyApplication/Model/APP_MyApplication_/DTC/GetBit4 ==
  note: GetBit
  u : Inport
  SEL : Inport  Port=2
  LoopOverBits : Subsystem
  y : Outport
  wires:
  u/1 -> LoopOverBits/1(u)
  SEL/1 -> LoopOverBits/2(SEL)
  LoopOverBits/1(y) -> y/1

== system APP_MyApplication/Model/APP_MyApplication_/DTC/GetBit5 ==
  note: GetBit
  u : Inport
  SEL : Inport  Port=2
  LoopOverBits : Subsystem
  y : Outport
  wires:
  u/1 -> LoopOverBits/1(u)
  SEL/1 -> LoopOverBits/2(SEL)
  LoopOverBits/1(y) -> y/1

== system APP_MyApplication/Model/APP_MyApplication_/DTC/GetBit6 ==
  note: GetBit
  u : Inport
  SEL : Inport  Port=2
  LoopOverBits : Subsystem
  y : Outport
  wires:
  u/1 -> LoopOverBits/1(u)
  SEL/1 -> LoopOverBits/2(SEL)
  LoopOverBits/1(y) -> y/1

== system APP_MyApplication/Model/APP_MyApplication_/DTC/OR ==
  note: OR
  u1 : Inport  OutDataTypeStr=boolean
  u2 : Inport  Port=2  OutDataTypeStr=boolean
  DataType : DataTypeConversion  OutDataTypeStr=boolean
  Operator : Logic  Operator=OR  AllPortsSameDT=off  OutDataTypeStr=boolean
  y : Outport
  wires:
  Operator/1 -> DataType/1
  u1/1 -> Operator/1
  u2/1 -> Operator/2
  DataType/1 -> y/1

== system APP_MyApplication/Model/APP_MyApplication_/DTC/OR1 ==
  note: OR
  u1 : Inport  OutDataTypeStr=boolean
  u2 : Inport  Port=2  OutDataTypeStr=boolean
  DataType : DataTypeConversion  OutDataTypeStr=boolean
  Operator : Logic  Operator=OR  AllPortsSameDT=off  OutDataTypeStr=boolean
  y : Outport
  wires:
  Operator/1 -> DataType/1
  u1/1 -> Operator/1
  u2/1 -> Operator/2
  DataType/1 -> y/1

== system APP_MyApplication/Model/APP_MyApplication_/DTC/OR2 ==
  note: OR
  u1 : Inport  OutDataTypeStr=boolean
  u2 : Inport  Port=2  OutDataTypeStr=boolean
  DataType : DataTypeConversion  OutDataTypeStr=boolean
  Operator : Logic  Operator=OR  AllPortsSameDT=off  OutDataTypeStr=boolean
  y : Outport
  wires:
  Operator/1 -> DataType/1
  u1/1 -> Operator/1
  u2/1 -> Operator/2
  DataType/1 -> y/1

== system APP_MyApplication/Model/APP_MyApplication_/DTC/OR3 ==
  note: OR
  u1 : Inport  OutDataTypeStr=boolean
  u2 : Inport  Port=2  OutDataTypeStr=boolean
  DataType : DataTypeConversion  OutDataTypeStr=boolean
  Operator : Logic  Operator=OR  AllPortsSameDT=off  OutDataTypeStr=boolean
  y : Outport
  wires:
  Operator/1 -> DataType/1
  u1/1 -> Operator/1
  u2/1 -> Operator/2
  DataType/1 -> y/1

== system APP_MyApplication/Model/APP_MyApplication_/DTC List/OR1 ==
  note: OR
  u1 : Inport  OutDataTypeStr=boolean
  u2 : Inport  Port=2  OutDataTypeStr=boolean
  DataType : DataTypeConversion  OutDataTypeStr=boolean
  Operator : Logic  Operator=OR  AllPortsSameDT=off  OutDataTypeStr=boolean
  y : Outport
  wires:
  Operator/1 -> DataType/1
  u1/1 -> Operator/1
  u2/1 -> Operator/2
  DataType/1 -> y/1

== system APP_MyApplication/Model/APP_MyApplication_/DateTime/DateTimeAssemble ==
  note: DateTimeAssemble
  Year : Inport  OutDataTypeStr=uint16
  Month : Inport  Port=2  OutDataTypeStr=uint8
  Day : Inport  Port=3  OutDataTypeStr=uint8
  Hours : Inport  Port=4  OutDataTypeStr=uint8
  Minutes : Inport  Port=5  OutDataTypeStr=uint8
  Seconds : Inport  Port=6  OutDataTypeStr=uint8
  CheckIfInputIsValid : Subsystem
  ConvertToDateTime : Subsystem
  ConvertToNrOfDays : Subsystem
  DT : Outport  OutDataTypeStr=uint32
  ENO : Outport  Port=2  OutDataTypeStr=boolean
  wires:
  ConvertToNrOfDays/1(u16_NrOfDays) -> ConvertToDateTime/4(u16_NrOfDays)
  ConvertToDateTime/1(u32_DateTime) -> DT/1
  Seconds/1 -> CheckIfInputIsValid/1(u8_SecondsIn)
  Minutes/1 -> CheckIfInputIsValid/2(u8_MinutesIn)
  Hours/1 -> CheckIfInputIsValid/3(u8_HoursIn)
  Day/1 -> CheckIfInputIsValid/4(u8_DayIn)
  Month/1 -> CheckIfInputIsValid/5(u8_MonthIn)
  Year/1 -> CheckIfInputIsValid/6(u16_YearIn)
  CheckIfInputIsValid/6(u16_Year) -> ConvertToNrOfDays/3(u16_Year)
  CheckIfInputIsValid/5(u8_Month) -> ConvertToNrOfDays/2(u8_Month)
  CheckIfInputIsValid/4(u8_Day) -> ConvertToNrOfDays/1(u8_Day)
  CheckIfInputIsValid/3(u8_Hours) -> ConvertToDateTime/3(u8_Hours)
  CheckIfInputIsValid/2(u8_Minutes) -> ConvertToDateTime/2(u8_Minutes)
  CheckIfInputIsValid/1(u8_Seconds) -> ConvertToDateTime/1(u8_Seconds)
  CheckIfInputIsValid/7(bo_ENO) -> ENO/1

== system APP_MyApplication/Model/APP_MyApplication_/DateTime/DateTimeAssemble1 ==
  note: DateTimeAssemble
  Year : Inport  OutDataTypeStr=uint16
  Month : Inport  Port=2  OutDataTypeStr=uint8
  Day : Inport  Port=3  OutDataTypeStr=uint8
  Hours : Inport  Port=4  OutDataTypeStr=uint8
  Minutes : Inport  Port=5  OutDataTypeStr=uint8
  Seconds : Inport  Port=6  OutDataTypeStr=uint8
  CheckIfInputIsValid : Subsystem
  ConvertToDateTime : Subsystem
  ConvertToNrOfDays : Subsystem
  DT : Outport  OutDataTypeStr=uint32
  ENO : Outport  Port=2  OutDataTypeStr=boolean
  wires:
  ConvertToNrOfDays/1(u16_NrOfDays) -> ConvertToDateTime/4(u16_NrOfDays)
  ConvertToDateTime/1(u32_DateTime) -> DT/1
  Seconds/1 -> CheckIfInputIsValid/1(u8_SecondsIn)
  Minutes/1 -> CheckIfInputIsValid/2(u8_MinutesIn)
  Hours/1 -> CheckIfInputIsValid/3(u8_HoursIn)
  Day/1 -> CheckIfInputIsValid/4(u8_DayIn)
  Month/1 -> CheckIfInputIsValid/5(u8_MonthIn)
  Year/1 -> CheckIfInputIsValid/6(u16_YearIn)
  CheckIfInputIsValid/6(u16_Year) -> ConvertToNrOfDays/3(u16_Year)
  CheckIfInputIsValid/5(u8_Month) -> ConvertToNrOfDays/2(u8_Month)
  CheckIfInputIsValid/4(u8_Day) -> ConvertToNrOfDays/1(u8_Day)
  CheckIfInputIsValid/3(u8_Hours) -> ConvertToDateTime/3(u8_Hours)
  CheckIfInputIsValid/2(u8_Minutes) -> ConvertToDateTime/2(u8_Minutes)
  CheckIfInputIsValid/1(u8_Seconds) -> ConvertToDateTime/1(u8_Seconds)
  CheckIfInputIsValid/7(bo_ENO) -> ENO/1

== system APP_MyApplication/Model/APP_MyApplication_/DateTime/DateTimeDisassemble ==
  note: Output
  note: Maximum
  note: Current
  note: Add 1970 years
  note: DateTimeDisassemble
  DT : Inport  OutDataTypeStr=uint32
  Add : Sum  OutDataTypeStr=uint32
  Add1 : Sum  OutDataTypeStr=uint16
  Add4 : Sum  OutDataTypeStr=uint8
  Bus Creator : BusCreator  Inputs='u8_Seconds','u8_Minutes','u8_Hours','u8_Day','u8_Month','u16_Year','u8_DayOfWeek'
  Bus Creator1 : BusCreator  Inputs=7
  Bus Selector : BusSelector  OutputSignals=u8_Seconds,u8_Minutes,u8_Hours,u8_Day,u8_Month,u16_Year,u8_DayOfWeek
  CheckIfTimeDataIsValid : Subsystem
  CheckLeapYearsAndRemainingDays : Subsystem
  Constant : Constant  OutDataTypeStr=uint8
  Constant1 : Constant  Value=1970  OutDataTypeStr=uint16
  Constant10 : Constant  Value=2099  OutDataTypeStr=uint16
  Constant11 : Constant  Value=12  OutDataTypeStr=uint8
  Constant12 : Constant  Value=31  OutDataTypeStr=uint8
  Constant13 : Constant  Value=4  OutDataTypeStr=uint8
  Constant7 : Constant  Value=59  OutDataTypeStr=uint8
  Constant8 : Constant  Value=59  OutDataTypeStr=uint8
  Constant9 : Constant  Value=23  OutDataTypeStr=uint8
  ConvertToDayOfWeek : Subsystem
  ConvertToMonthAndDay : Subsystem  TreatAsAtomicUnit=on
  ConvertToTimeAndNrOfDays : Subsystem
  Data Type Conversion1 : DataTypeConversion  OutDataTypeStr=uint8
  Switch : Switch  Criteria=u2 ~= 0
  Year : Outport  OutDataTypeStr=uint16
  Month : Outport  Port=2  OutDataTypeStr=uint8
  Day : Outport  Port=3  OutDataTypeStr=uint8
  Hours : Outport  Port=4  OutDataTypeStr=uint8
  Minutes : Outport  Port=5  OutDataTypeStr=uint8
  Seconds : Outport  Port=6  OutDataTypeStr=uint8
  DayOfWeek : Outport  Port=7  OutDataTypeStr=uint8
  ENO : Outport  Port=8  OutDataTypeStr=boolean
  wires:
  Add1/1 -> Bus Creator/6  "u16_Year"
  ConvertToTimeAndNrOfDays/1(u8_Seconds) -> Bus Creator/1  "u8_Seconds"
  ConvertToTimeAndNrOfDays/3(u8_Hours) -> Bus Creator/3  "u8_Hours"
  ConvertToTimeAndNrOfDays/2(u8_Minutes) -> Bus Creator/2  "u8_Minutes"
  ConvertToMonthAndDay/2(u16_DayMinusOne) -> Add/1
  CheckLeapYearsAndRemainingDays/2(u16_Year) -> Add1/1
  Constant1/1 -> Add1/2
  CheckLeapYearsAndRemainingDays/3(bo_LeapYear) -> ConvertToMonthAndDay/2(bo_LeapYear)
  DT/1 -> CheckIfTimeDataIsValid/1(u32_DateTime), ConvertToTimeAndNrOfDays/1(u32_DateTime)
  Add/1 -> Data Type Conversion1/1
  ConvertToMonthAndDay/1(u8_MonthMinusOne) -> Add4/1
  Add4/1 -> Bus Creator/5  "u8_Month"
  Bus Selector/1 -> Seconds/1  "<u8_Seconds>"
  Bus Selector/2 -> Minutes/1  "<u8_Minutes>"
  Bus Selector/3 -> Hours/1  "<u8_Hours>"
  Bus Selector/5 -> Month/1  "<u8_Month>"
  Bus Creator/1 -> Switch/1  "st_CurrDateTime"
  Switch/1 -> Bus Selector/1  "st_OutDateTime"
  Bus Creator1/1 -> Switch/3  "st_MaxDataTime"
  Constant7/1 -> Bus Creator1/1  "u8_Seconds"
  Constant8/1 -> Bus Creator1/2  "u8_Minutes"
  Constant9/1 -> Bus Creator1/3  "u8_Hours"
  Constant11/1 -> Bus Creator1/5  "u8_Month"
  Constant13/1 -> Bus Creator1/7  "u8_DayOfWeek"
  Bus Selector/4 -> Day/1  "<u8_Day>"
  Data Type Conversion1/1 -> Bus Creator/4  "u8_Day"
  Bus Selector/6 -> Year/1  "<u16_Year>"
  Constant12/1 -> Bus Creator1/4  "u8_Day"
  Constant10/1 -> Bus Creator1/6  "u16_Year"
  Bus Selector/7 -> DayOfWeek/1  "<u8_DayOfWeek>"
  ConvertToTimeAndNrOfDays/4(u16_NrOfDays) -> ConvertToDayOfWeek/1(u16_NrOfDays), CheckLeapYearsAndRemainingDays/1(u16_NrOfDays)
  Constant/1 -> Add4/2, Add/2
  ConvertToDayOfWeek/1(u8_DayOfWeek) -> Bus Creator/7  "u8_DayOfWeek"
  CheckLeapYearsAndRemainingDays/1(u16_TempDate) -> ConvertToMonthAndDay/1(u16_TempDate)
  CheckIfTimeDataIsValid/1(bo_ENO) -> ENO/1, Switch/2

== system APP_MyApplication/Model/APP_MyApplication_/EEProm/EnabledSubsystem ==
  In1 : Inport
  Enable : EnablePort  InitFcn=|
      | try
      |    MBDS_BlockCallback('Update', gcb);
      | end
      settings: AttributesFormatString=States when enabling: %<StatesWhenEnabling>
  Out1 : Outport
      settings: AttributesFormatString=Output when disabled: %<OutputWhenDisabled>
  wires:
  In1/1 -> Out1/1

== system APP_MyApplication/Model/APP_MyApplication_/EEProm/EnabledSubsystem1 ==
  "In1 " : Inport
  In2 : Inport  Port=2
  Enable : EnablePort  InitFcn=|
      | try
      |    MBDS_BlockCallback('Update', gcb);
      | end
      settings: AttributesFormatString=States when enabling: %<StatesWhenEnabling>
  out_NVMModelRelatedData.NVMVariables2.StoreVariablesToNVM : KIBES_Signal/KIBES_Signal  MBDS_LibraryBlock=on  DatabaseKey=440  SignalName=NVMModelRelatedData.NVMVariables2.StoreVariablesToNVM  SymbolName=NVMModelRelatedData_NVMVariables2_StoreVariablesToNVM_000440  DataType=boolean  Init=0  Slope=1  Bias=0  DataSize=1  fpDataType=boolean  BlockIOType=Outport  DeviceType=0
  out_NVMVariables2.Var2 : KIBES_Signal/KIBES_Signal  MBDS_LibraryBlock=on  DatabaseKey=437  SignalName=NVMVariables2.Var2  SymbolName=NVMVariables2_Var2_000437  DataType=uint32  Init=0  Slope=1  Bias=0  DataSize=1  fpDataType=uint32  BlockIOType=Outport  DeviceType=0
  wires:
  "In1 "/1 -> out_NVMVariables2.Var2/1
  In2/1 -> out_NVMModelRelatedData.NVMVariables2.StoreVariablesToNVM/1

== system APP_MyApplication/Model/APP_MyApplication_/EEProm/EnabledSubsystem2 ==
  In1 : Inport
  Enable : EnablePort  InitFcn=|
      | try
      |    MBDS_BlockCallback('Update', gcb);
      | end
      settings: AttributesFormatString=States when enabling: %<StatesWhenEnabling>
  Out1 : Outport
      settings: AttributesFormatString=Output when disabled: %<OutputWhenDisabled>
  wires:
  In1/1 -> Out1/1
